simulink model "model_following_position_ref"  (R2023b)
settings: Solver=FixedStepDiscrete  StartTime=0.0  StopTime=mf_cfg.stop_time  FixedStep=mf_cfg.Ts_ref  RelTol=1e-3
values from neighbouring files (symbols this model uses):
  mf_cfg = evalin('base', 'mf_cfg')    [run_study.m]
settings Model: Creator=user  LastModifiedBy=user
settings DataIOCC: SaveFormat=StructureWithTime

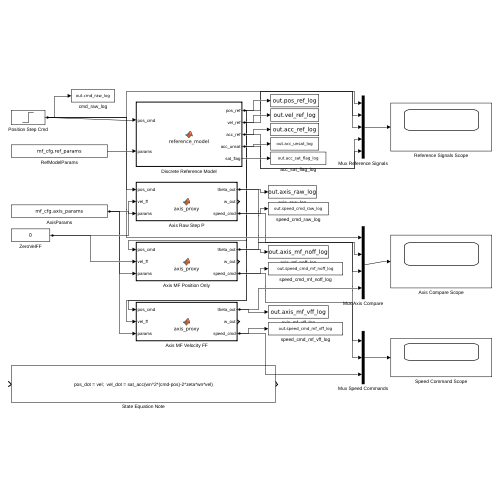
[thumbnail: Simulink's stored preview of the top-level diagram]
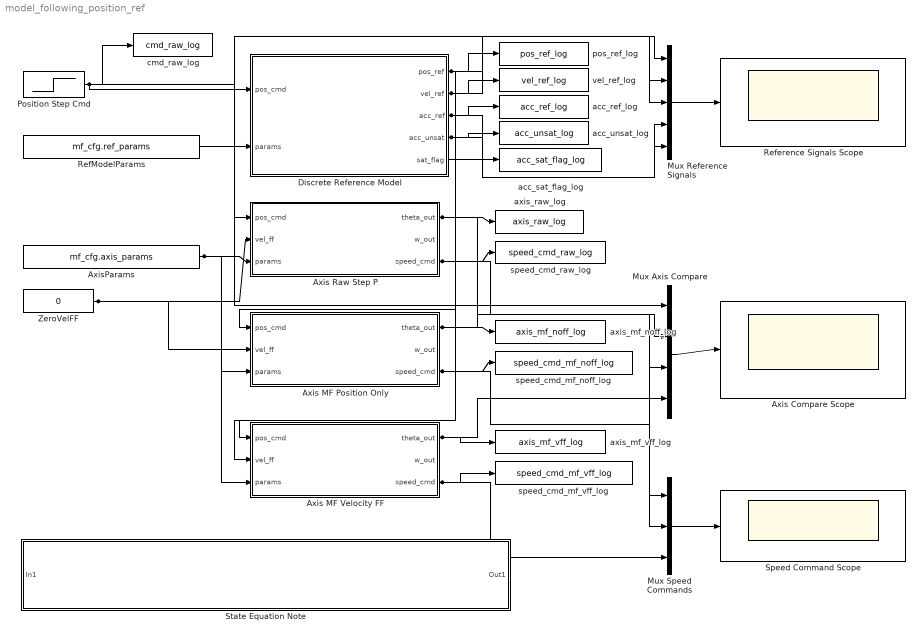
== system model_following_position_ref ==
  Axis Compare Scope : Scope
  Axis MF Position Only : MATLAB Function  TreatAsAtomicUnit=on
  Axis MF Velocity FF : MATLAB Function  TreatAsAtomicUnit=on
  Axis Raw Step P : MATLAB Function  TreatAsAtomicUnit=on
  AxisParams : Constant  Value=mf_cfg.axis_params
  Discrete Reference Model : MATLAB Function  TreatAsAtomicUnit=on
  Mux Axis Compare : Mux
  Mux Reference Signals : Mux  Inputs=5
  Mux Speed Commands : Mux  Inputs=3
  Position Step Cmd : Step  Time=mf_cfg.step_time  After=mf_cfg.step_rad  SampleTime=mf_cfg.Ts_ref
  RefModelParams : Constant  Value=mf_cfg.ref_params
  Reference Signals Scope : Scope
  Speed Command Scope : Scope
  State Equation Note : Subsystem
      mask Display: disp('pos_dot = vel;  vel_dot = sat_acc(wn^2*(cmd-pos)-2*zeta*wn*vel)')
  ZeroVelFF : Constant  Value=0
  acc_ref_log : ToWorkspace  VariableName=acc_ref_log  SaveFormat=Structure With Time  SampleTime=-1
  acc_sat_flag_log : ToWorkspace  VariableName=acc_sat_flag_log  SaveFormat=Structure With Time  SampleTime=-1
  acc_unsat_log : ToWorkspace  VariableName=acc_unsat_log  SaveFormat=Structure With Time  SampleTime=-1
  axis_mf_noff_log : ToWorkspace  VariableName=axis_mf_noff_log  SaveFormat=Structure With Time  SampleTime=-1
  axis_mf_vff_log : ToWorkspace  VariableName=axis_mf_vff_log  SaveFormat=Structure With Time  SampleTime=-1
  axis_raw_log : ToWorkspace  VariableName=axis_raw_log  SaveFormat=Structure With Time  SampleTime=-1
  cmd_raw_log : ToWorkspace  VariableName=cmd_raw_log  SaveFormat=Structure With Time  SampleTime=-1
  pos_ref_log : ToWorkspace  VariableName=pos_ref_log  SaveFormat=Structure With Time  SampleTime=-1
  speed_cmd_mf_noff_log : ToWorkspace  VariableName=speed_cmd_mf_noff_log  SaveFormat=Structure With Time  SampleTime=-1
  speed_cmd_mf_vff_log : ToWorkspace  VariableName=speed_cmd_mf_vff_log  SaveFormat=Structure With Time  SampleTime=-1
  speed_cmd_raw_log : ToWorkspace  VariableName=speed_cmd_raw_log  SaveFormat=Structure With Time  SampleTime=-1
  vel_ref_log : ToWorkspace  VariableName=vel_ref_log  SaveFormat=Structure With Time  SampleTime=-1
  wires:
  Position Step Cmd/1 -> Discrete Reference Model/1(pos_cmd), cmd_raw_log/1, Axis Raw Step P/1(pos_cmd), Mux Reference Signals/1, Mux Axis Compare/1
  RefModelParams/1 -> Discrete Reference Model/2(params)
  Discrete Reference Model/1(pos_ref) -> pos_ref_log/1, Axis MF Position Only/1(pos_cmd), Axis MF Velocity FF/1(pos_cmd), Mux Reference Signals/2
  Discrete Reference Model/2(vel_ref) -> vel_ref_log/1, Axis MF Velocity FF/2(vel_ff), Mux Reference Signals/3
  Discrete Reference Model/3(acc_ref) -> acc_ref_log/1, Mux Reference Signals/4
  Discrete Reference Model/4(acc_unsat) -> acc_unsat_log/1, Mux Reference Signals/5
  Discrete Reference Model/5(sat_flag) -> acc_sat_flag_log/1
  ZeroVelFF/1 -> Axis Raw Step P/2(vel_ff), Axis MF Position Only/2(vel_ff)
  AxisParams/1 -> Axis Raw Step P/3(params), Axis MF Position Only/3(params), Axis MF Velocity FF/3(params)
  Axis Raw Step P/1(theta_out) -> axis_raw_log/1, Mux Axis Compare/2
  Axis MF Position Only/1(theta_out) -> axis_mf_noff_log/1, Mux Axis Compare/3
  Axis MF Velocity FF/1(theta_out) -> axis_mf_vff_log/1, Mux Axis Compare/4
  Axis Raw Step P/3(speed_cmd) -> speed_cmd_raw_log/1, Mux Speed Commands/1
  Axis MF Position Only/3(speed_cmd) -> speed_cmd_mf_noff_log/1, Mux Speed Commands/2
  Axis MF Velocity FF/3(speed_cmd) -> speed_cmd_mf_vff_log/1, Mux Speed Commands/3
  Mux Reference Signals/1 -> Reference Signals Scope/1
  Mux Axis Compare/1 -> Axis Compare Scope/1
  Mux Speed Commands/1 -> Speed Command Scope/1

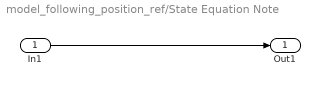
== system model_following_position_ref/State Equation Note ==
  In1 : Inport
  Out1 : Outport
  wires:
  In1/1 -> Out1/1

== matlab function model_following_position_ref/Axis Raw Step P ==
  data: pos_cmd input; theta_out output; vel_ff input; params input; w_out output; speed_cmd output
function [theta_out, w_out, speed_cmd] = axis_proxy(pos_cmd, vel_ff, params)
% Discrete position loop + velocity feedforward + first-order speed loop.
% params = [pos_kp, vel_ff_gain, speed_tau, Ts, speed_limit]
persistent theta w
if isempty(theta)
    theta = 0;
    w = 0;
end

pos_kp = params(1);
vel_ff_gain = params(2);
speed_tau = max(params(3), eps);
Ts = params(4);
speed_limit = abs(params(5));

speed_cmd_unsat = pos_kp * (pos_cmd - theta) + vel_ff_gain * vel_ff;
speed_cmd = min(max(speed_cmd_unsat, -speed_limit), speed_limit);
w = w + (speed_cmd - w) * Ts / speed_tau;
theta = theta + w * Ts;

theta_out = theta;
w_out = w;
end

== matlab function model_following_position_ref/Discrete Reference Model ==
  data: pos_cmd input; pos_ref output; params input; vel_ref output; acc_ref output; acc_unsat output; sat_flag output
function [pos_ref, vel_ref, acc_ref, acc_unsat, sat_flag] = reference_model(pos_cmd, params)
% Discrete saturated second-order reference model.
% params = [wn, zeta, Ts, acc_limit, vel_limit]
persistent pos vel
if isempty(pos)
    pos = 0;
    vel = 0;
end

wn = params(1);
zeta = params(2);
Ts = params(3);
acc_limit = abs(params(4));
vel_limit = abs(params(5));

acc_unsat = wn * wn * (pos_cmd - pos) - 2 * zeta * wn * vel;
acc_limited = min(max(acc_unsat, -acc_limit), acc_limit);

vel_candidate = vel + acc_limited * Ts;
vel_next = min(max(vel_candidate, -vel_limit), vel_limit);
acc_ref = (vel_next - vel) / Ts;
pos_next = pos + vel_next * Ts;

sat_flag = double(abs(acc_unsat - acc_ref) > 1e-9 || abs(vel_candidate - vel_next) > 1e-9);

pos = pos_next;
vel = vel_next;
pos_ref = pos;
vel_ref = vel;
end

== matlab function model_following_position_ref/Axis MF Position Only ==
  data: pos_cmd input; theta_out output; vel_ff input; params input; w_out output; speed_cmd output
function [theta_out, w_out, speed_cmd] = axis_proxy(pos_cmd, vel_ff, params)
% Discrete position loop + velocity feedforward + first-order speed loop.
% params = [pos_kp, vel_ff_gain, speed_tau, Ts, speed_limit]
persistent theta w
if isempty(theta)
    theta = 0;
    w = 0;
end

pos_kp = params(1);
vel_ff_gain = params(2);
speed_tau = max(params(3), eps);
Ts = params(4);
speed_limit = abs(params(5));

speed_cmd_unsat = pos_kp * (pos_cmd - theta) + vel_ff_gain * vel_ff;
speed_cmd = min(max(speed_cmd_unsat, -speed_limit), speed_limit);
w = w + (speed_cmd - w) * Ts / speed_tau;
theta = theta + w * Ts;

theta_out = theta;
w_out = w;
end

== matlab function model_following_position_ref/Axis MF Velocity FF ==
  data: pos_cmd input; theta_out output; vel_ff input; params input; w_out output; speed_cmd output
function [theta_out, w_out, speed_cmd] = axis_proxy(pos_cmd, vel_ff, params)
% Discrete position loop + velocity feedforward + first-order speed loop.
% params = [pos_kp, vel_ff_gain, speed_tau, Ts, speed_limit]
persistent theta w
if isempty(theta)
    theta = 0;
    w = 0;
end

pos_kp = params(1);
vel_ff_gain = params(2);
speed_tau = max(params(3), eps);
Ts = params(4);
speed_limit = abs(params(5));

speed_cmd_unsat = pos_kp * (pos_cmd - theta) + vel_ff_gain * vel_ff;
speed_cmd = min(max(speed_cmd_unsat, -speed_limit), speed_limit);
w = w + (speed_cmd - w) * Ts / speed_tau;
theta = theta + w * Ts;

theta_out = theta;
w_out = w;
end
